simulink model "fake_theta"  (R2013a)
settings: Solver=ode45  StartTime=0.0  StopTime=1000  RelTol=1e-3
undefined symbols (not defined in the file or in its folder): zz
libraries: simulink x1
settings Model: Creator=Leo  LastModifiedBy=Leo

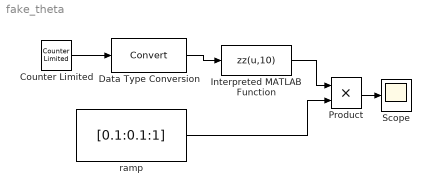
== system fake_theta ==
  " ramp" : Constant  Value=[0.1:0.1:1]
  Counter Limited : simulink/Sources/Counter Limited  uplimit=9  tsamp=10
  Data Type Conversion : DataTypeConversion
  Interpreted MATLAB Function : MATLABFcn  MATLABFcn=zz(u,10)
  Product : Product
  Scope : Scope
  wires:
  Counter Limited/1 -> Data Type Conversion/1
  Interpreted MATLAB Function/1 -> Product/1
  " ramp"/1 -> Product/2
  Product/1 -> Scope/1
  Data Type Conversion/1 -> Interpreted MATLAB Function/1
